simulink model "actividad3"  (R2019a)
settings: Solver=VariableStepAuto  StartTime=0.0  StopTime=1000.0  RelTol=1e-3
libraries: simulink x4
settings Model: Creator=pon_c  LastModifiedBy=pon_c

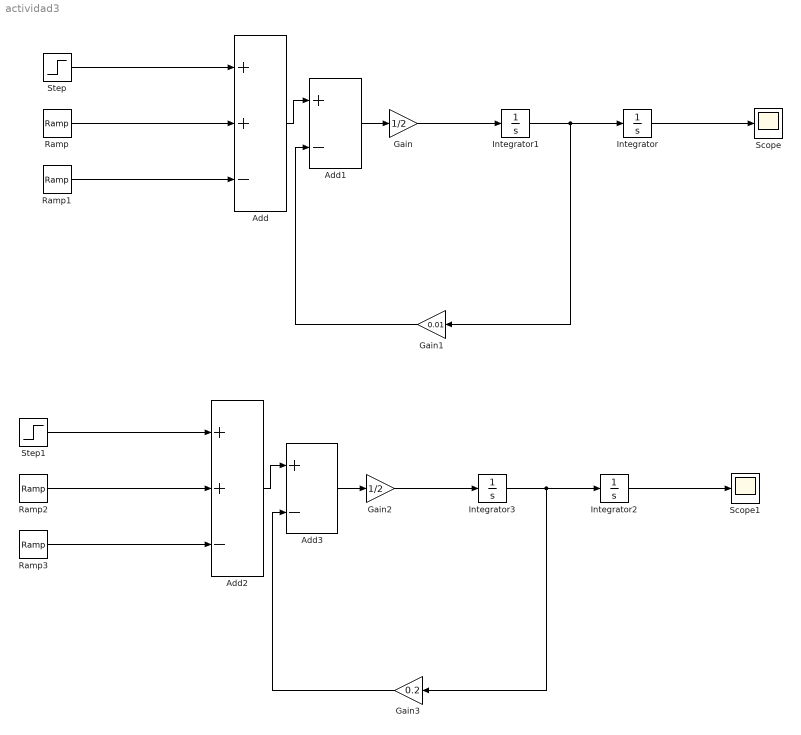
== system actividad3 ==
  Add : Sum  Inputs=++-
  Add1 : Sum  Inputs=+-
  Add2 : Sum  Inputs=++-
  Add3 : Sum  Inputs=+-
  Gain : Gain  Gain=1/2
  Gain1 : Gain  Gain=0.01
  Gain2 : Gain  Gain=1/2
  Gain3 : Gain  Gain=0.2
  Integrator{,1..3} (4 alike) : Integrator
  Ramp : simulink/Sources/Ramp  slope=100  start=1  InitialOutput=0
  Ramp1 : simulink/Sources/Ramp  slope=100  start=1.1  InitialOutput=0
  Ramp2 : simulink/Sources/Ramp  slope=100  start=1  InitialOutput=0
  Ramp3 : simulink/Sources/Ramp  slope=100  start=1.1  InitialOutput=0
  Scope : Scope
  Scope1 : Scope
  Step : Step  Time=1.1  After=-10  SampleTime=0
  Step1 : Step  Time=1.1  After=-10  SampleTime=0
  wires:
  Step/1 -> Add/1
  Ramp/1 -> Add/2
  Ramp1/1 -> Add/3
  Add/1 -> Add1/1
  Gain/1 -> Integrator1/1
  Integrator1/1 -> Gain1/1, Integrator/1
  Integrator/1 -> Scope/1
  Gain1/1 -> Add1/2
  Add1/1 -> Gain/1
  Gain3/1 -> Add3/2
  Gain2/1 -> Integrator3/1
  Step1/1 -> Add2/1
  Ramp2/1 -> Add2/2
  Ramp3/1 -> Add2/3
  Integrator3/1 -> Gain3/1, Integrator2/1
  Add3/1 -> Gain2/1
  Add2/1 -> Add3/1
  Integrator2/1 -> Scope1/1
